simulink model "Part3_3"  (R2022a)
settings: Solver=VariableStepAuto  StartTime=0.0  StopTime=10  RelTol=1e-3
values from neighbouring files (symbols this model uses):
  D = diag([0.01, 0.01, 0.01])    [Driver_3.m]    (also in Driver_3NL.m)
  g = [0,0,-9.81]    [Driver_3.m]    (also in Driver_3NL.m)
  g2 = [0,0,0,-9.81]    [Driver_3.m]    (also in Driver_3NL.m)
  I_tf = diag([3e-6, 3e-6, 1e-5, 1])    [Driver_3.m]    (also in Driver_3NL.m)
  In = inv(I)    [Driver_3.m]    (also in Driver_3NL.m)
  k = 0.01    [Driver_3.m]    (also in Driver_3NL.m)
  K_d = 0.8    [Driver_3.m]    (also in Driver_3NL.m)
  K_i = 0.1    [Driver_3.m]    (also in Driver_3NL.m)
  K_p = 1.5    [Driver_3.m]    (also in Driver_3NL.m)
  m = 0.5    [Driver_3.m]    (also in Driver_3NL.m)
  mvec = [1 ... (first row only)    [Driver_3.m]    (also in Driver_3NL.m)
  TF = diag(tf)    [Driver_3.m]
  TF2 = inv(tf2)    [Driver_3.m]    (also in Driver_3NL.m)
  tf_34 = [L*k, 0, -L*k, 0 ... (first row only)    [Driver_3.m]    (also in Driver_3NL.m)
  w0 = sqrt(9.81*m/(4*k))    [Driver_3.m]    (also in Driver_3NL.m)
undefined symbols (not defined in the file or in its folder): K_dxy, K_ixy, K_pxy, tf_xy, uxy, uzp
settings Model: Creator=askeo  LastModifiedBy=askeo

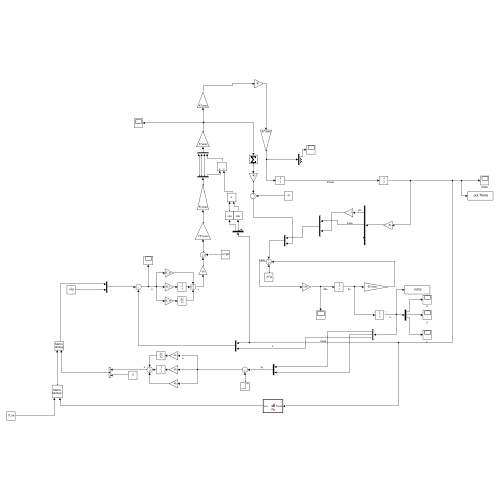
[thumbnail: Simulink's stored preview of the top-level diagram]
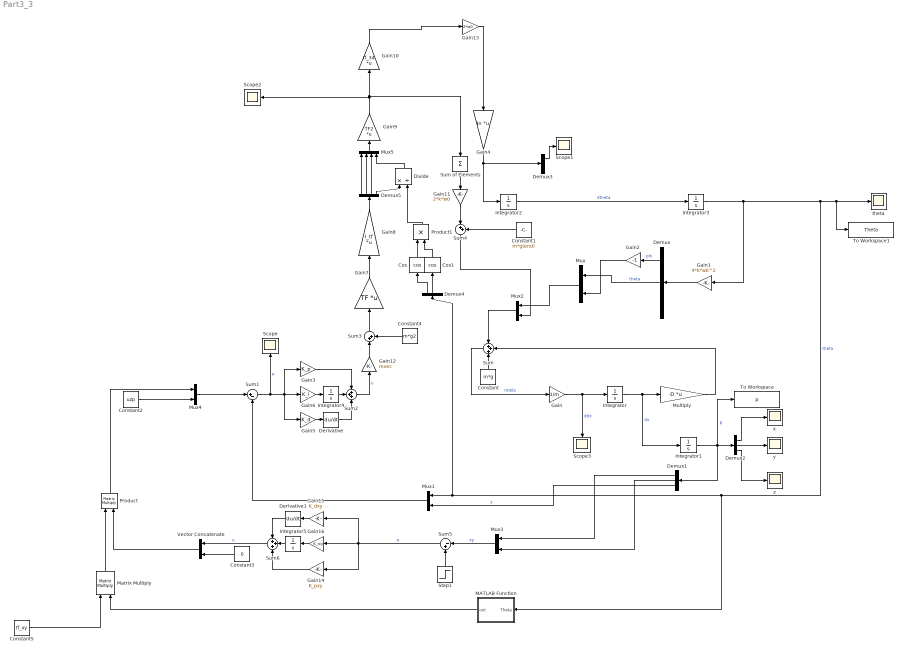
== system Part3_3 ==
  Constant : Constant  Value=m*g
  Constant1 : Constant  Value=m*g(end)
  Constant2 : Constant  Value=uzp
  Constant3 : Constant  Value=0
  Constant4 : Constant  Value=m*g2
  Constant5 : Constant  Value=tf_xy  VectorParams1D=off
  Cos : Trigonometry  Operator=cos
  Cos1 : Trigonometry  Operator=cos
  Demux{,1..4} (5 alike) : Demux  Outputs=3
  Demux5 : Demux
  Derivative : Derivative
  Derivative1 : Derivative
  Divide : Product  Inputs=*/
  Gain : Gain  Gain=1/m
  Gain1 : Gain  Gain=4*k*w0^2
  Gain10 : Gain  Gain=tf_34  Multiplication=Matrix(K*u) (u vector)
  Gain11 : Gain  Gain=2*k*w0
  Gain12 : Gain  Gain=mvec
  Gain13 : Gain  Gain=2*w0
  Gain14 : Gain  Gain=K_pxy
  Gain15 : Gain  Gain=K_dxy
  Gain16 : Gain  Gain=K_ixy
  Gain2 : Gain  Gain=-1
  Gain3 : Gain  Gain=K_p
  Gain4 : Gain  Gain=In  Multiplication=Matrix(K*u) (u vector)
  Gain5 : Gain  Gain=K_d
  Gain6 : Gain  Gain=K_i
  Gain7 : Gain  Gain=TF  Multiplication=Matrix(K*u) (u vector)
  Gain8 : Gain  Gain=I_tf  Multiplication=Matrix(K*u) (u vector)
  Gain9 : Gain  Gain=TF2  Multiplication=Matrix(K*u) (u vector)
  Integrator : Integrator  InitialCondition=[0;0;0]
  Integrator1 : Integrator  InitialCondition=[0;0;0]
  Integrator2 : Integrator  InitialCondition=[0;0;0]
  Integrator3 : Integrator  InitialCondition=[0; 0; 0]
  Integrator4 : Integrator
  Integrator5 : Integrator
  MATLAB Function : MATLAB Function  TreatAsAtomicUnit=on
  Matrix Multiply : Product  Multiplication=Matrix(*)
  Multiply : Gain  Gain=-D  Multiplication=Matrix(K*u) (u vector)
  Mux{,1..4} (5 alike) : Mux  Inputs=2
  Mux5 : Mux
  Product : Product  Multiplication=Matrix(*)
  Product1 : Product
  Scope{,1..3} (4 alike) : Scope
  Step1 : Step  Time=0  After=uxy  SampleTime=0
  Sum : Sum  Inputs=+++
  Sum of Elements : Sum  Inputs=+
  Sum1 : Sum  Inputs=|+-
  Sum2 : Sum  Inputs=+++
  Sum3 : Sum  Inputs=|++
  Sum4 : Sum  Inputs=|++
  Sum5 : Sum  Inputs=|-+
  Sum6 : Sum  Inputs=+++
  To Workspace : ToWorkspace  VariableName=p  SampleTime=-1
  To Workspace1 : ToWorkspace  VariableName=Theta  SampleTime=0.001
  Vector Concatenate : Concatenate
  theta : Scope
  x : Scope
  y : Scope
  z : Scope
  wires:
  Constant1/1 -> Sum4/2
  Sum/1 -> Gain/1  "mddx"
  Gain11/1 -> Sum4/1
  Gain2/1 -> Mux/2
  Gain12/1 -> Sum3/1
  Demux2/3 -> z/1
  Demux1/3 -> Mux1/2  "z"
  Sum3/1 -> Gain7/1
  Integrator4/1 -> Sum2/2
  Constant4/1 -> Sum3/2
  Gain9/1 -> Gain10/1, Sum of Elements/1, Scope2/1
  Sum of Elements/1 -> Gain11/1
  Sum4/1 -> Mux2/2
  Gain7/1 -> Gain8/1
  Derivative/1 -> Sum2/3
  Gain5/1 -> Derivative/1
  Integrator2/1 -> Integrator3/1  "dtheta"
  Demux/1 -> Gain2/1  "phi"
  Mux1/1 -> Sum1/2
  Demux/2 -> Mux/1  "theta"
  Integrator/1 -> Integrator1/1, Multiply/1  "dx"
  Mux/1 -> Mux2/1
  Sum2/1 -> Gain12/1  "u"
  Sum1/1 -> Gain5/1, Gain6/1, Gain3/1, Scope/1  "e"
  Demux3/1 -> Scope1/1
  Gain6/1 -> Integrator4/1
  Gain1/1 -> Demux/1
  Mux2/1 -> Sum/1
  Gain13/1 -> Gain4/1
  Integrator1/1 -> Demux1/1, Demux2/1, To Workspace/1  "p"
  Gain3/1 -> Sum2/1
  Constant/1 -> Sum/3
  Gain/1 -> Scope3/1, Integrator/1  "ddx"
  Multiply/1 -> Sum/2
  Gain4/1 -> Integrator2/1, Demux3/1
  Gain10/1 -> Gain13/1
  Demux1/1 -> Mux3/1
  Demux1/2 -> Mux3/2
  Mux3/1 -> Sum5/1  "xy"
  Step1/1 -> Sum5/2
  Gain16/1 -> Integrator5/1
  Sum5/1 -> Gain15/1, Gain16/1, Gain14/1  "e"
  Integrator5/1 -> Sum6/2
  Gain15/1 -> Derivative1/1
  Derivative1/1 -> Sum6/1
  Gain14/1 -> Sum6/3
  Mux4/1 -> Sum1/1
  Constant2/1 -> Mux4/2
  Sum6/1 -> Vector Concatenate/1  "u"
  Constant3/1 -> Vector Concatenate/2
  Integrator3/1 -> Gain1/1, MATLAB Function/1(Theta), Mux1/1, Demux4/1, To Workspace1/1, theta/1  "theta"
  Demux2/2 -> y/1
  Demux2/1 -> x/1
  MATLAB Function/1(out) -> Matrix Multiply/2
  Product/1 -> Mux4/1
  Vector Concatenate/1 -> Product/2
  Matrix Multiply/1 -> Product/1
  Constant5/1 -> Matrix Multiply/1
  Demux4/2 -> Cos1/1
  Demux4/1 -> Cos/1
  Cos1/1 -> Product1/2
  Cos/1 -> Product1/1
  Gain8/1 -> Demux5/1
  Demux5/4 -> Divide/1
  Product1/1 -> Divide/2
  Divide/1 -> Mux5/4
  Mux5/1 -> Gain9/1
  Demux5/3 -> Mux5/3
  Demux5/2 -> Mux5/2
  Demux5/1 -> Mux5/1

== matlab function Part3_3/MATLAB Function ==
  data: Theta input; out output
function out = Rb(Theta)

phi = Theta(1);
theta = Theta(2);
psi = Theta(3);

rbi = [cos(psi)*cos(theta), cos(psi)*sin(theta)*sin(phi) - sin(psi)*cos(phi), sin(psi)*sin(phi) + cos(psi)*sin(theta)*cos(phi)
    sin(psi)*cos(theta), cos(psi)*cos(phi) + sin(psi)*sin(theta)*sin(phi), sin(psi)*sin(theta)*sin(phi) - cos(psi)*sin(phi)
    -sin(theta), cos(theta)*sin(phi), cos(theta)*cos(phi)];

out = rbi;
end
